simulink model "Task1Aa"  (R2024a)
settings: Solver=VariableStepAuto  StartTime=0.0  StopTime=10.0  RelTol=1e-3
undefined symbols (not defined in the file): b, k, m
settings Model: Creator=kyleo  LastModifiedBy=kyleo

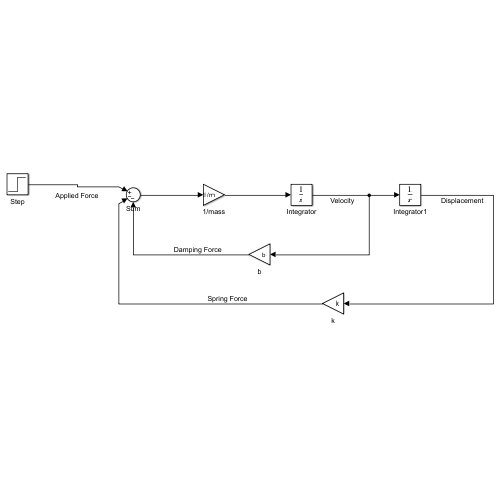
[thumbnail: Simulink's stored preview of the top-level diagram]
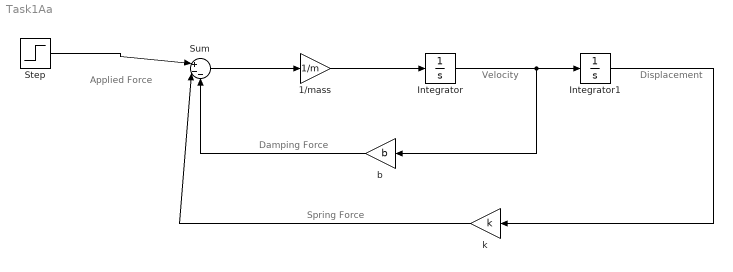
== system Task1Aa ==
  note: Displacement
  note: Velocity
  note: Spring Force
  note: Damping Force
  note: Applied Force
  1/mass : Gain  Gain=1/m
  Integrator : Integrator
  Integrator1 : Integrator
  Step : Step  SampleTime=0
  Sum : Sum  Inputs=|+--
  b : Gain  Gain=b
  k : Gain  Gain=k
  wires:
  Sum/1 -> 1/mass/1
  1/mass/1 -> Integrator/1
  Integrator/1 -> b/1, Integrator1/1
  Integrator1/1 -> k/1
  k/1 -> Sum/2
  b/1 -> Sum/3
  Step/1 -> Sum/1
